simulink model "Boucle_fermee_sim"  (R2019a)
settings: Solver=VariableStepAuto  StartTime=0.0  StopTime=120  MaxStep=1e-2  MinStep=1e-3  RelTol=1e-3
values from neighbouring files (symbols this model uses):
  CorInt = tf(1 , [1 0])    [TP6.m]
  CorPD = tf([Td 1] , 1)*Kp    [TP6.m]
libraries: cstblocks x2
settings Model: Creator=fereka231  LastModifiedBy=fereka231
settings SolverCC: InitialStep=1e-3

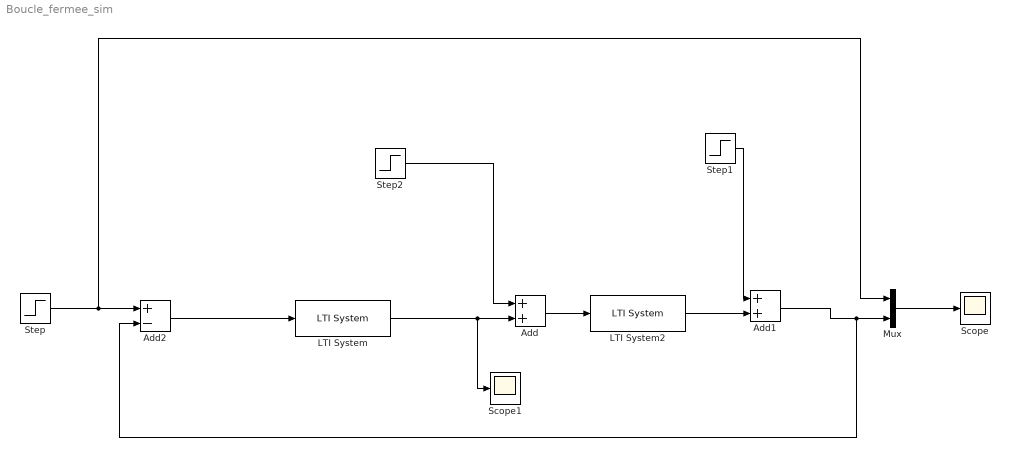
== system Boucle_fermee_sim ==
  Add : Sum
  Add1 : Sum
  Add2 : Sum  Inputs=+-
  LTI System : cstblocks/LTI System  sys=CorInt*CorPD  IC=[]
  LTI System2 : cstblocks/LTI System  sys=G  IC=[]
  Mux : Mux  Inputs=2
  Scope : Scope
  Scope1 : Scope
  Step : Step  After=0.5  SampleTime=0
  Step1 : Step  Time=60  After=0.5  SampleTime=0
  Step2 : Step  Time=30  After=0.5  SampleTime=0
  wires:
  Step/1 -> Mux/1, Add2/1
  Step2/1 -> Add/1
  Add/1 -> LTI System2/1
  LTI System2/1 -> Add1/2
  Step1/1 -> Add1/1
  Mux/1 -> Scope/1
  Add1/1 -> Add2/2, Mux/2
  Add2/1 -> LTI System/1
  LTI System/1 -> Scope1/1, Add/2
